simulink model "Ejer2_SDR (1)"  (R2023b)
settings: Solver=VariableStepAuto  StartTime=0.0  StopTime=10.0  RelTol=1e-3
undefined symbols (not defined in the file): startfcn_spectrum_analyzer
libraries: dspmlti4 x2, dspsnks4 x1, rtlsdr_book_library x1, sdrrlib x1
settings Model: Creator=katty  LastModifiedBy=katty

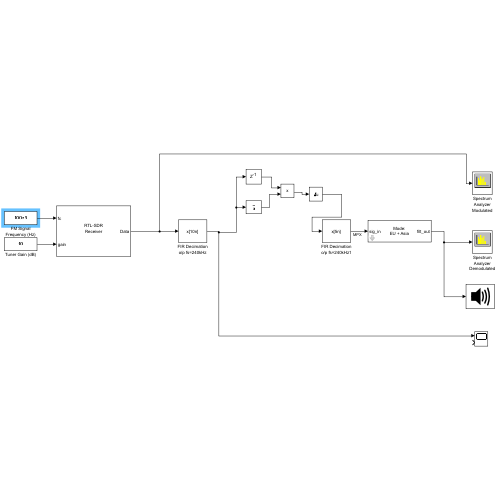
[thumbnail: Simulink's stored preview of the top-level diagram]
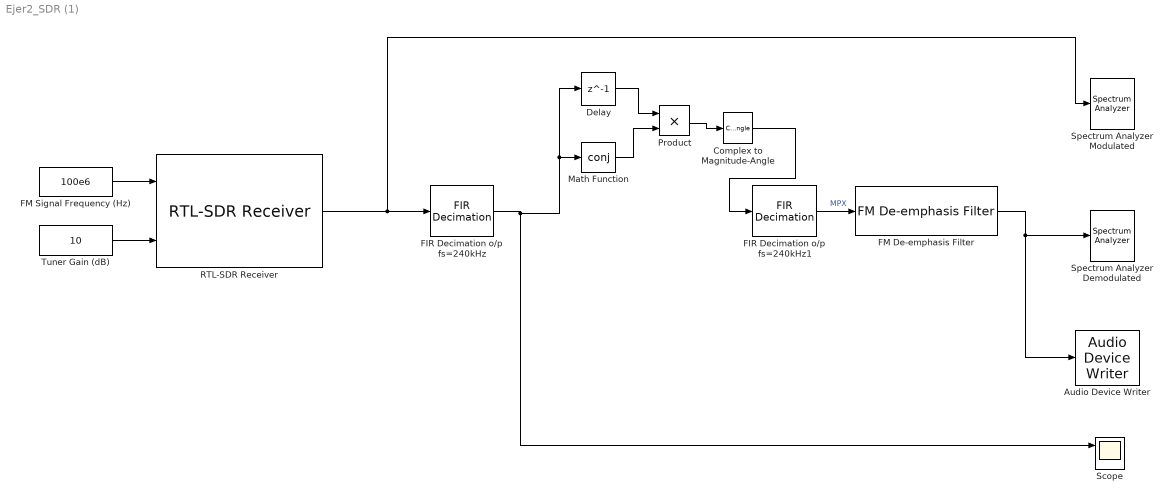
== system Ejer2_SDR (1) ==
  Audio Device Writer : dspsnks4/Audio Device Writer  Driver=DirectSound  Device=Default  InheritSampleRate=on  SampleRate=44100  BitDepth=16-bit integer  BufferSize=4096  NumBuffers=10  DefaultOutputChannelMapping=on  OutputChannelMapping=1:2  OutputNumUnderrunSamples=off  DriverIdx=1  DeviceWarnFlag=''
  Complex to Magnitude-Angle : ComplexToMagnitudeAngle  Output=Angle
  Delay : Delay  DelayLength=1  InitialCondition=0
  FIR Decimation o/p fs=240kHz : dspmlti4/FIR Decimation  FilterSource=Dialog parameters  h=firpm(50, [0 120e3 240e3 (2.4e6/2)]/(2.4e6/2), [1 1 0 0], [1 1],20)  D=10  filtStruct=Direct form  FilterObject=Hm_firdecim  InputProcessing=Columns as channels (frame based)  framing=Allow multirate processing  AllowArbitraryInputLength=off  inputOffset=0  outputBufInitCond=0  roundingMode=Floor  overflowMode=off  firstCoeffDataTypeStr=Inherit: Same word length as input  firstCoeffMin=[]  firstCoeffMax=[]  firstCoeffLastDataTypeStr=Inherit: Same word length as input  outputDataTypeStr=Inherit: Same as accumulator  outputMin=[]  outputMax=[]  outputLastDataTypeStr=Inherit: Same as accumulator
  FIR Decimation o/p fs=240kHz1 : dspmlti4/FIR Decimation  FilterSource=Dialog parameters  h=firpm(50, [0 120e3 240e3 (2.4e6/2)]/(2.4e6/2), [1 1 0 0], [1 1],20)  D=5  filtStruct=Direct form  FilterObject=Hm_firdecim  InputProcessing=Columns as channels (frame based)  framing=Allow multirate processing  AllowArbitraryInputLength=off  inputOffset=0  outputBufInitCond=0  roundingMode=Floor  overflowMode=off  firstCoeffDataTypeStr=Inherit: Same word length as input  firstCoeffMin=[]  firstCoeffMax=[]  firstCoeffLastDataTypeStr=Inherit: Same word length as input  outputDataTypeStr=Inherit: Same as accumulator  outputMin=[]  outputMax=[]  outputLastDataTypeStr=Inherit: Same as accumulator
  FM De-emphasis Filter : rtlsdr_book_library/FM Demod Tools/FM De-emphasis Filter  region=Europe, Asia  fs=48e3
      settings: SourceProductName=RTL-SDR Book Library
  FM Signal Frequency (Hz) : Constant  Value=100e6
  Math Function : Math  Operator=conj  SignedPower=on
  Product : Product
  RTL-SDR Receiver : sdrrlib/RTL-SDR Receiver  IPAddress=0  CenterFrequencySource=Input port  CenterFrequency=102.5e6  GainSource=Input port  Gain=0  ADCRate=2e6  FrequencyCorrection=0  LostSamplesOutputPort=off  LatencyOutputPort=off  OutputDataType=int16  FrameLength=1024  EnableBurstMode=off  NumFramesInBurst=20  sobjType=sdrr.internal.SDRRTLReceiverSL  dataUDPPort=-1  ctrlUDPPort=-1  subDeviceList=nosubdev  sdrBlockType=SDRBlockTypeSLT.SDRRxBlock  requester=UNUSED_BY_SFCN  sdrExecutionMode=SDRExecutionModeSLT.ExecModeHW  BypassUserLogic=off  DecimatorSelect=DDC decimator  SourceSelect=RF data  SineAmplitude=16000  EnableInternalClock=off  BypassIQBalance=off  IFBandwidth=40e6  ADCRateSource=Dialog  IntermediateFrequency=0  DecimationFactorSource=Dialog  DecimationFactor=512  RFFrequencyIsTunable=logical(1)  SampleTime=(1024)/(2e6)  IFBandwidthSource=Dialog  SineFrequency=30000  BypassDCBlockingFilter=off  IntermediateFrequencySource=Dialog  IQBalanceCoefficients=64  SkipAllHardwareResetAndInitialization=off  EnableIQCalibrationTable=on  CacheIQCalibrationTable=off  EnableOffsetTuning=off  EnableRTLAGC=off  EnableTestMode=off  EnableTunerAGC=off  FrequencyCorrectionSource=Dialog  NumMLBuffers=128  NumUSBBuffers=16  RTLCrystalFrequency=28800000  TunerCrystalFrequency=28800000
  Scope : Scope  NumInputPorts=2
  Spectrum Analyzer Demodulated : SpectrumAnalyzer  StartFcn=startfcn_spectrum_analyzer;  WindowPosition=[1084 622 778 262]  ScopeFrameLocation=window  Method=Welch  SampleRate=48000  AxesScaling=Manual  Span=400000  StartFrequency=-200000  StopFrequency=200000  AveragingMethod=Running  YLabel=dBm  YLimits=[-90,25]  ColorLimits=[-145.27268916534743,20]  ShowGrid=off  ShowLegend=on  DefaultConfigurationName=spbscopes.SpectrumAnalyzerBlockCfg
  Spectrum Analyzer Modulated : SpectrumAnalyzer  StartFcn=startfcn_spectrum_analyzer;  WindowPosition=[528.000000,212.000000,778.000000,225.000000,]  ScopeFrameLocation=window  Method=Welch  SampleRate=240000  AxesScaling=Manual  Span=400000  StartFrequency=-200000  StopFrequency=200000  AveragingMethod=Running  YLabel=dBm  YLimits=[-69.383930992470468,32.02048051388072]  ColorLimits=[-145.27268916534743,20]  ShowGrid=off  DefaultConfigurationName=spbscopes.SpectrumAnalyzerBlockCfg
  Tuner Gain (dB) : Constant  Value=10
  wires:
  RTL-SDR Receiver/1 -> Spectrum Analyzer Modulated/1, FIR Decimation o/p fs=240kHz/1
  FIR Decimation o/p fs=240kHz1/1 -> FM De-emphasis Filter/1  "MPX"
  FM De-emphasis Filter/1 -> Audio Device Writer/1, Spectrum Analyzer Demodulated/1
  Tuner Gain (dB)/1 -> RTL-SDR Receiver/2
  FM Signal Frequency (Hz)/1 -> RTL-SDR Receiver/1
  Math Function/1 -> Product/2
  FIR Decimation o/p fs=240kHz/1 -> Delay/1, Math Function/1, Scope/1
  Complex to Magnitude-Angle/1 -> FIR Decimation o/p fs=240kHz1/1
  Product/1 -> Complex to Magnitude-Angle/1
  Delay/1 -> Product/1
